simulink model "hw2_q1"  (R2020a)
settings: Solver=VariableStepAuto  StartTime=0.0  StopTime=0.07  RelTol=1e-3
libraries: powerlib x14
settings Model: Creator=tahsi  LastModifiedBy=tahsi
settings DebuggingCC: UnconnectedInputMsg=none  UnconnectedOutputMsg=none  UnconnectedLineMsg=none
settings ModelReferenceCC: EnableRefExpFcnMdlSchedulingChecks=off
settings RTWCC: Description=Generic Real-Time Target

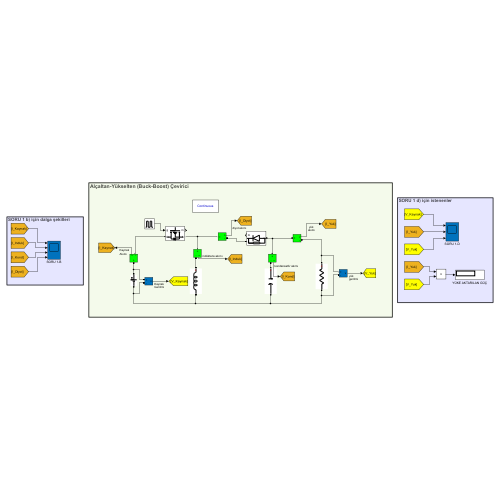
[thumbnail: Simulink's stored preview of the top-level diagram]
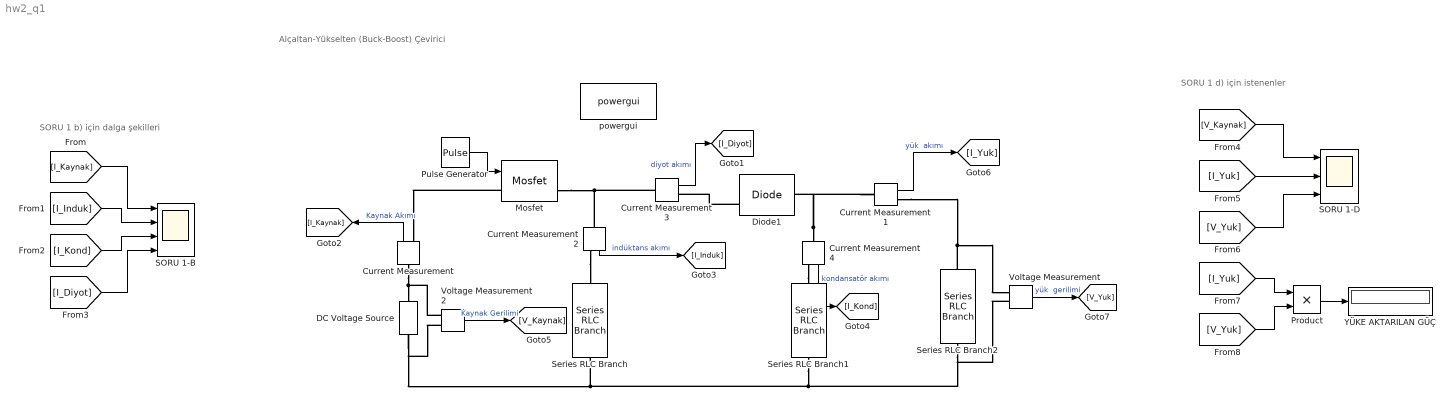
== system hw2_q1 ==
  note: Alçaltan-Yükselten (Buck-Boost) Çevirici
  note: SORU 1 b) için dalga şekilleri
  note: SORU 1 d) için istenenler
  Current Measurement{,1..4} (5 alike) : powerlib/Measurements/Current Measurement  PhasorSimulation=off  OutputType=Complex  PSBequivalent=0
  DC Voltage Source : powerlib/Electrical Sources/DC Voltage Source  Amplitude=48  Measurements=None
  Diode1 : powerlib/Power Electronics/Diode  Ron=0.001  Lon=0  Vf=0.8  IC=0  UseSnubber=0  Rs=500  Cs=250e-9  Measurements=on
  Mosfet : powerlib/Power Electronics/Mosfet  Ron=8e-3  Lon=0  Rd=0.0209  Vfd=1.3  IC=0  Rs=220000  Cs=inf  Measurements=on
  Product : Product
  Pulse Generator : DiscretePulseGenerator  PulseType=Time based  Period=1/40000  PulseWidth=25
  SORU 1-B : Scope  NumInputPorts=4
  SORU 1-D : Scope  NumInputPorts=3
  Series RLC Branch : powerlib/Elements/Series RLC Branch  LConnTagsString=__new0  RConnTagsString=__new0  BranchType=L  Resistance=0  Inductance=5e-3  SetiL0=off  InitialCurrent=0  Capacitance=0  Setx0=off  InitialVoltage=0  Measurements=None
  Series RLC Branch1 : powerlib/Elements/Series RLC Branch  LConnTagsString=__new0  RConnTagsString=__new0  BranchType=C  Resistance=1  Inductance=1e-3  SetiL0=off  InitialCurrent=0  Capacitance=100e-6  Setx0=off  InitialVoltage=20  Measurements=None
  Series RLC Branch2 : powerlib/Elements/Series RLC Branch  LConnTagsString=__new0  RConnTagsString=__new0  BranchType=R  Resistance=5  Inductance=0  SetiL0=off  InitialCurrent=0  Capacitance=0  Setx0=off  InitialVoltage=0  Measurements=None
  Voltage Measurement : powerlib/Measurements/Voltage Measurement  PhasorSimulation=off  OutputType=Complex  PSBequivalent=0
  Voltage Measurement2 : powerlib/Measurements/Voltage Measurement  PhasorSimulation=off  OutputType=Complex  PSBequivalent=0
  YÜKE AKTARILAN GÜÇ : Display
  powergui : powerlib/powergui  Priority=1  SimulationMode=Continuous  SampleTime=50e-6  frequency=60  Iterations=50  frequencyindice=0  Pbase=100e6  ErrMax=1e-4  UnitsV=kV  UnitsW=MW  buscounter=0  FunctionMessages=off  echomessages=off  EnableUseOfTLC=off  CurrentSourceSwitches=off  DisableSnubberDevices=off  DisableRonSwitches=off  DisableVfSwitches=off  DisplayEquations=off  AutomaticDiscreteSolvers=off  SolverType=Tustin/Backward Euler (TBE)  Interpol=off  ExternalGateDelay=off  methode=off  Ts=100  x0status=blocks  SPID=on  SwTol=0  HookPort=off  NonlinearTolerance=1e-4  nMaxIteration=100  ContinueOnMaxIteration=off  RestoreLinks=warning  ResistiveCurrentMeasurement=off  Frange=[0:2:500]  Ylog=off  Xlog=on  ShowGrid=off  save=off  variable=ZData  structure=0  ZoomFFT=off  StartTime=0.0  cycles=1  DisplayStyle=1  fundamental=60  FreqAxis=off  MaxFrequency=1000  frequencyindicesteady=1  RmsSteady=1  display=off
  wires:
  Current Measurement2/1 -> [I_Induk]  "indüktans akımı"
  Pulse Generator/1 -> Mosfet/1
  Current Measurement1/1 -> [I_Yuk]  "yük  akımı"
  Current Measurement3/1 -> [I_Diyot]  "diyot akımı"
  Current Measurement4/1 -> [I_Kond]  "kondansatör akımı"
  Voltage Measurement2/1 -> [V_Kaynak]  "Kaynak Gerilimi"
  Current Measurement/1 -> [I_Kaynak]  "Kaynak Akımı"
  Voltage Measurement/1 -> [V_Yuk]  "yük  gerilimi"
  [I_Kaynak] -> SORU 1-B/1
  [I_Induk] -> SORU 1-B/2
  [I_Kond] -> SORU 1-B/3
  [I_Diyot] -> SORU 1-B/4
  [V_Kaynak] -> SORU 1-D/1
  [I_Yuk] -> SORU 1-D/2
  [V_Yuk] -> SORU 1-D/3
  [I_Yuk] -> Product/1
  [V_Yuk] -> Product/2
  Product/1 -> YÜKE AKTARILAN GÜÇ/1
  connections:
  Current Measurement2/LConn1 -- Mosfet/RConn1 -- Current Measurement3/LConn1
  Series RLC Branch2/LConn1 -- Voltage Measurement/LConn1 -- Current Measurement1/RConn1
  Current Measurement/LConn1 -- Voltage Measurement2/LConn1 -- DC Voltage Source/RConn1
  Mosfet/LConn1 -- Current Measurement/RConn1
  Current Measurement2/RConn1 -- Series RLC Branch/LConn1
  Current Measurement4/RConn1 -- Series RLC Branch1/LConn1
  Series RLC Branch1/RConn1 -- Voltage Measurement/LConn2 -- Series RLC Branch2/RConn1 -- Voltage Measurement2/LConn2 -- DC Voltage Source/LConn1 -- Series RLC Branch/RConn1
  Current Measurement4/LConn1 -- Diode1/LConn1 -- Current Measurement1/LConn1
  Diode1/RConn1 -- Current Measurement3/RConn1
